simulink model "carSim"  (Simulink 10.2)
settings: Solver=ode23tb  StartTime=0.0  StopTime=10  FixedStep=1e-3  MaxStep=1e-2  RelTol=1e-3  EnableMultiTasking=on
libraries: simulink x1
settings Model: Creator=hp  LastModifiedBy=11634
settings SolverCC: AlgebraicLoopSolver=LineSearch
settings DataIOCC: LimitDataPoints=on  SignalLoggingName=sigsOut
settings OptimizationCC: ExpressionDepthLimit=2147483647  InitFltsAndDblsToZero=on
settings DebuggingCC: SaveWithParameterizedLinksMsg=none  SignalResolutionControl=TryResolveAllWithWarning  MultiTaskDSMMsg=warning  MultiTaskCondExecSysMsg=none  StateNameClashWarn=warning
settings HardwareCC: TargetUnknown=on
settings GRTTargetCC: TargetFcnLib=ansi_tfl_tmw.mat

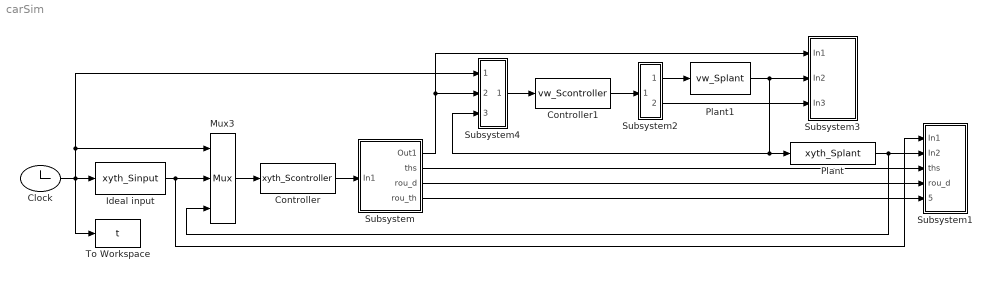
== system carSim ==
  Clock : Clock
  Controller : S-Function  FunctionName=xyth_Scontroller  SFunctionDeploymentMode=off  EnableBusSupport=off
  Controller1 : S-Function  FunctionName=vw_Scontroller  SFunctionDeploymentMode=off  EnableBusSupport=off
  Ideal input : S-Function  FunctionName=xyth_Sinput  SFunctionDeploymentMode=off  EnableBusSupport=off
  Mux3 : Mux  Inputs=3
  Plant : S-Function  FunctionName=xyth_Splant  SFunctionDeploymentMode=off  EnableBusSupport=off
  Plant1 : S-Function  FunctionName=vw_Splant  SFunctionDeploymentMode=off  EnableBusSupport=off
  Subsystem : Subsystem
  Subsystem1 : Subsystem
  Subsystem2 : Subsystem
  Subsystem3 : Subsystem
  Subsystem4 : Subsystem
  To Workspace : ToWorkspace  VariableName=t  SampleTime=-1
  wires:
  Plant/1 -> Mux3/3, Subsystem1/2(In2)
  Clock/1 -> Subsystem4/1(In1), Mux3/1, Ideal input/1, To Workspace/1
  Mux3/1 -> Controller/1
  Ideal input/1 -> Mux3/2, Subsystem1/1(In1)
  Controller/1 -> Subsystem/1(In1)
  Subsystem/2(ths) -> Subsystem1/3(ths)
  Subsystem/3(rou_d) -> Subsystem1/4(rou_d)
  Subsystem/4(rou_th) -> Subsystem1/5(rou_th)
  Plant1/1 -> Subsystem3/2(In2), Plant/1, Subsystem4/3(In2)
  Controller1/1 -> Subsystem2/1(In1)
  Subsystem2/1(Out1) -> Plant1/1
  Subsystem/1(Out1) -> Subsystem3/1(In1), Subsystem4/2(In3)
  Subsystem4/1(Out1) -> Controller1/1
  Subsystem2/2(Out3) -> Subsystem3/3(In3)

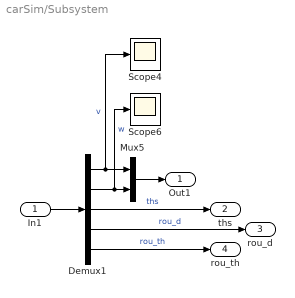
== system carSim/Subsystem ==
  In1 : Inport
  Demux1 : Demux  Outputs=5
  Mux5 : Mux  Inputs=2
  Scope4 : Scope
  Scope6 : Scope
  Out1 : Outport
  ths : Outport  Port=2
  rou_d : Outport  Port=3
  rou_th : Outport  Port=4
  wires:
  In1/1 -> Demux1/1
  Demux1/2 -> Scope6/1, Mux5/2  "w"
  Mux5/1 -> Out1/1
  Demux1/1 -> Scope4/1, Mux5/1  "v"
  Demux1/3 -> ths/1  "ths"
  Demux1/4 -> rou_d/1  "rou_d"
  Demux1/5 -> rou_th/1  "rou_th"

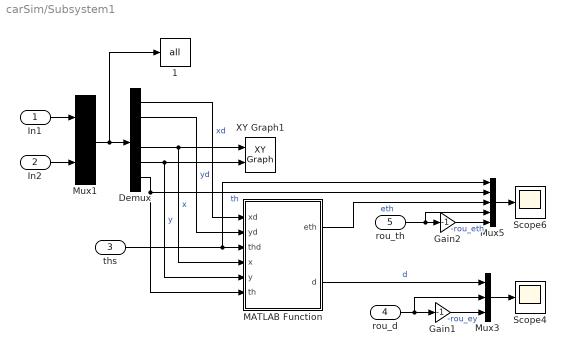
== system carSim/Subsystem1 ==
  In1 : Inport
  In2 : Inport  Port=2
  ths : Inport  Port=3
  rou_d : Inport  Port=4
  rou_th : Inport  Port=5
  " 1" : ToWorkspace  VariableName=all  SampleTime=-1
  Demux : Demux  Outputs=6
  Gain1 : Gain  Gain=-1
  Gain2 : Gain  Gain=-1
  MATLAB Function : MATLAB Function  TreatAsAtomicUnit=on
  Mux1 : Mux  Inputs=2
  Mux3 : Mux  Inputs=3
  Mux5 : Mux  Inputs=5
  Scope4 : Scope
  Scope6 : Scope
  XY Graph1 : simulink/Sinks/XY Graph  xmin=-4  xmax=4  ymin=-4  ymax=4  st=-1
  wires:
  Demux/1 -> MATLAB Function/1(xd)  "xd"
  Demux/5 -> XY Graph1/2, MATLAB Function/5(y)  "y"
  Mux1/1 -> Demux/1, " 1"/1
  rou_th/1 -> Mux5/4, Gain2/1
  Gain2/1 -> Mux5/5  "-rou_eth"
  rou_d/1 -> Gain1/1, Mux3/2
  Demux/4 -> XY Graph1/1, MATLAB Function/4(x)  "x"
  Demux/2 -> MATLAB Function/2(yd)  "yd"
  Demux/6 -> MATLAB Function/6(th), Mux5/2  "th"
  MATLAB Function/1(eth) -> Mux5/3  "eth"
  In2/1 -> Mux1/2
  Gain1/1 -> Mux3/3  "-rou_ey"
  MATLAB Function/2(d) -> Mux3/1  "d"
  In1/1 -> Mux1/1
  ths/1 -> Mux5/1, MATLAB Function/3(thd)
  Mux3/1 -> Scope4/1
  Mux5/1 -> Scope6/1

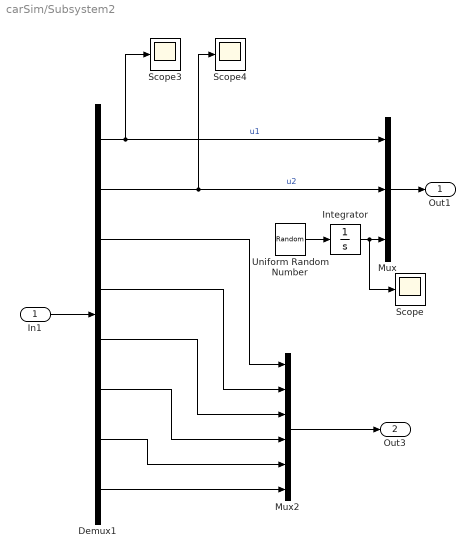
== system carSim/Subsystem2 ==
  In1 : Inport
  Demux1 : Demux  Outputs=8
  Integrator : Integrator
  Mux : Mux  Inputs=3
  Mux2 : Mux  Inputs=6
  Scope : Scope
  Scope3 : Scope
  Scope4 : Scope
  Uniform Random Number : UniformRandomNumber  SampleTime=0.1
  Out1 : Outport
  Out3 : Outport  Port=2
  wires:
  Demux1/1 -> Scope3/1, Mux/1  "u1"
  Demux1/2 -> Scope4/1, Mux/2  "u2"
  In1/1 -> Demux1/1
  Mux/1 -> Out1/1
  Demux1/5 -> Mux2/3
  Demux1/3 -> Mux2/1
  Demux1/4 -> Mux2/2
  Mux2/1 -> Out3/1
  Demux1/8 -> Mux2/6
  Demux1/7 -> Mux2/5
  Demux1/6 -> Mux2/4
  Uniform Random Number/1 -> Integrator/1
  Integrator/1 -> Scope/1, Mux/3

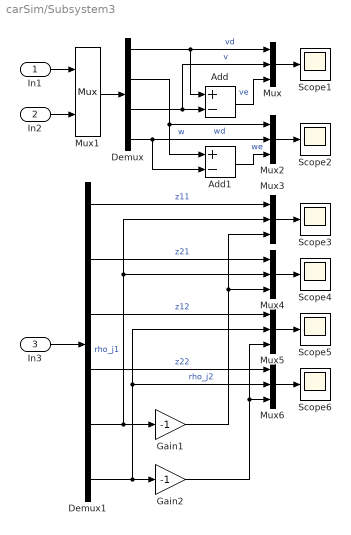
== system carSim/Subsystem3 ==
  In1 : Inport
  In2 : Inport  Port=2
  In3 : Inport  Port=3
  Add : Sum  Inputs=+-
  Add1 : Sum  Inputs=+-
  Demux : Demux
  Demux1 : Demux  Outputs=6
  Gain1 : Gain  Gain=-1
  Gain2 : Gain  Gain=-1
  Mux{,2..6} (6 alike) : Mux  Inputs=3
  Mux1 : Mux  Inputs=2
  Scope{1..6} (6 alike) : Scope
  wires:
  Add1/1 -> Mux2/3  "we"
  Demux/2 -> Add1/1, Mux2/1  "wd"
  Mux2/1 -> Scope2/1
  In1/1 -> Mux1/1
  Mux1/1 -> Demux/1
  Demux/4 -> Add1/2, Mux2/2  "w"
  Add/1 -> Mux/3  "ve"
  Mux/1 -> Scope1/1
  Demux/3 -> Mux/2, Add/2  "v"
  Demux/1 -> Add/1, Mux/1  "vd"
  In3/1 -> Demux1/1
  Mux3/1 -> Scope3/1
  Demux1/5 -> Mux4/2, Mux3/2, Gain1/1  "rho_j1"
  Demux1/6 -> Mux6/2, Mux5/2, Gain2/1  "rho_j2"
  Demux1/1 -> Mux3/1  "z11"
  Mux4/1 -> Scope4/1
  Mux5/1 -> Scope5/1
  Mux6/1 -> Scope6/1
  Demux1/2 -> Mux4/1  "z21"
  Demux1/3 -> Mux5/1  "z12"
  Demux1/4 -> Mux6/1  "z22"
  Gain1/1 -> Mux4/3, Mux3/3
  Gain2/1 -> Mux6/3, Mux5/3
  In2/1 -> Mux1/2

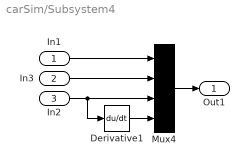
== system carSim/Subsystem4 ==
  In1 : Inport
  In3 : Inport  Port=2
  In2 : Inport  Port=3
  Derivative1 : Derivative
  Mux4 : Mux
  Out1 : Outport
  wires:
  Mux4/1 -> Out1/1
  Derivative1/1 -> Mux4/4
  In3/1 -> Mux4/2
  In2/1 -> Derivative1/1, Mux4/3
  In1/1 -> Mux4/1

== matlab function Subsystem1/MATLAB Function ==
  data: xd input double; yd input double; thd input double; x input double; y input double; th input double; eth output double; d output double
function [eth,d] = VLyapunov(xd,yd,thd,x,y,th)
xIe=xd-x;
yIe=yd-y;
eth=thNormalization(th-thd);
d = sqrt(xIe^2+yIe^2);
